simulink model "DCMotor1b"  (R2021b)
settings: Solver=VariableStepAuto  StartTime=0.0  StopTime=10.0  RelTol=1e-3
undefined symbols (not defined in the file): b, denB, J, K, L, numB, R
settings Model: Creator=feyzi  LastModifiedBy=feyzi

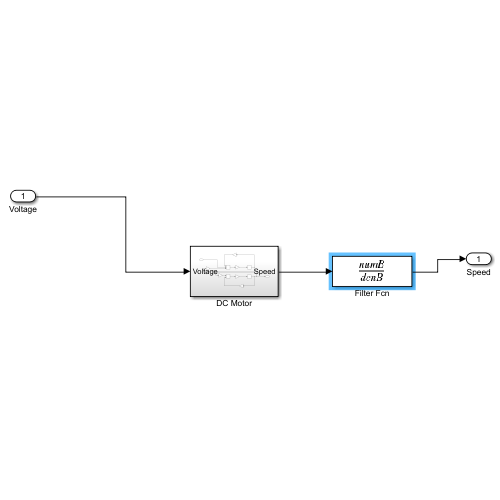
[thumbnail: Simulink's stored preview of the top-level diagram]
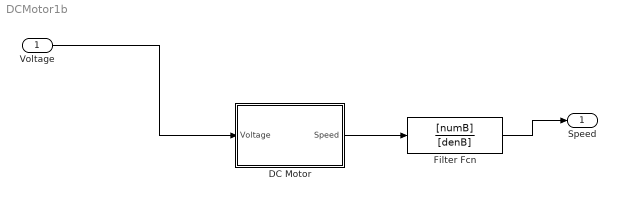
== system DCMotor1b ==
  Voltage : Inport
  DC Motor : Subsystem
  Filter Fcn : TransferFcn  Numerator=[numB]  Denominator=[denB]
  Speed : Outport
  wires:
  Voltage/1 -> DC Motor/1(Voltage)
  Filter Fcn/1 -> Speed/1
  DC Motor/1(Speed) -> Filter Fcn/1

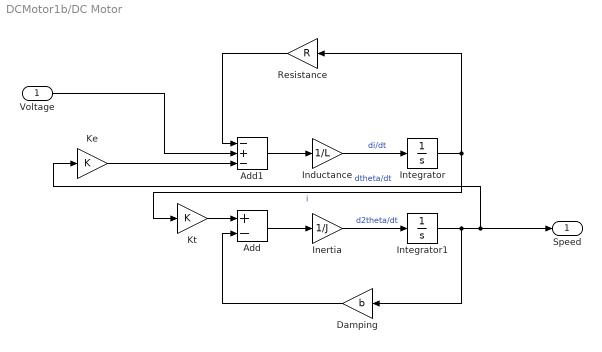
== system DCMotor1b/DC Motor ==
  Voltage : Inport
  Add : Sum  Inputs=+-
  Add1 : Sum  Inputs=-+-
  Damping : Gain  Gain=b
  Inductance : Gain  Gain=1/L
  Inertia : Gain  Gain=1/J
  Integrator : Integrator
  Integrator1 : Integrator
  Ke : Gain  Gain=K
  Kt : Gain  Gain=K
  Resistance : Gain  Gain=R
  Speed : Outport
  wires:
  Resistance/1 -> Add1/1
  Add/1 -> Inertia/1
  Inertia/1 -> Integrator1/1  "d2theta/dt"
  Integrator1/1 -> Speed/1, Ke/1, Damping/1  "dtheta/dt"
  Add1/1 -> Inductance/1
  Voltage/1 -> Add1/2
  Inductance/1 -> Integrator/1  "di/dt"
  Kt/1 -> Add/1
  Damping/1 -> Add/2
  Integrator/1 -> Resistance/1, Kt/1  "i"
  Ke/1 -> Add1/3
